simulink model "ECE371_Lab6_Exact"  (R2017a)
settings: Solver=ode3  StartTime=0.0  StopTime=Tf  FixedStep=0.01  RelTol=1e-3
values from neighbouring files (symbols this model uses):
  Rp = 6    [ECE371_Lab6_matlab.m]
  Rs = 0.05    [ECE371_Lab6_matlab.m]
libraries: simulink x1
settings Model: Creator=localmgr  LastModifiedBy=localmgr

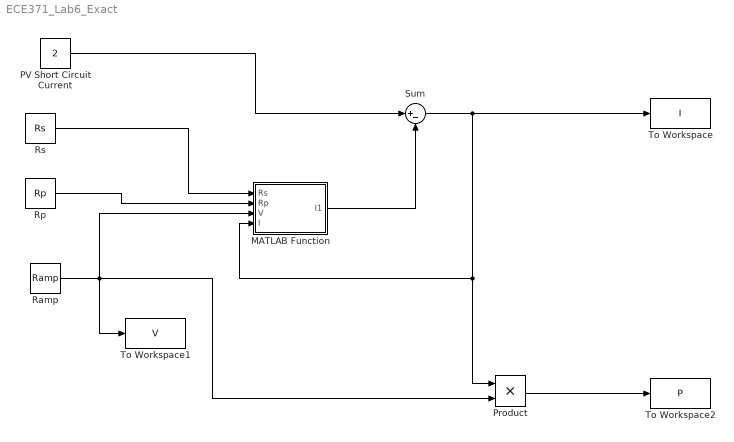
== system ECE371_Lab6_Exact ==
  MATLAB Function : MATLAB Function  TreatAsAtomicUnit=on
  PV Short Circuit Current : Constant  Value=2
  Product : Product
  Ramp : simulink/Sources/Ramp  slope=1  start=0  X0=0
  Rp : Constant  Value=Rp
  Rs : Constant  Value=Rs
  Sum : Sum  Inputs=|+-
  To Workspace : ToWorkspace  VariableName=I  SampleTime=-1
  To Workspace1 : ToWorkspace  VariableName=V  SampleTime=-1
  To Workspace2 : ToWorkspace  VariableName=P  SampleTime=-1
  wires:
  PV Short Circuit Current/1 -> Sum/1
  Sum/1 -> To Workspace/1, MATLAB Function/4(I), Product/1
  Ramp/1 -> To Workspace1/1, MATLAB Function/3(V), Product/2
  Product/1 -> To Workspace2/1
  Rs/1 -> MATLAB Function/1(Rs)
  Rp/1 -> MATLAB Function/2(Rp)
  MATLAB Function/1(I1) -> Sum/2

== matlab function ECE371_Lab6_Exact/MATLAB Function ==
  data: Rs input; I1 output; Rp input; V input; I input
function I1 = fcn(Rs, Rp, V,I)

I1 = 1e-9*(exp(38.927*(V+I*Rs))-1)+(V+I*Rs)/Rp;
